simulink model "test03_mod02_firmware_removed"  (Simulink 7.3)
settings: Solver=FixedStepDiscrete  SolverMode=SingleTasking  StartTime=0.0  StopTime=inf  FixedStep=0.01  RelTol=1e-3  SampleTimeConstraint=Specified
undefined symbols (not defined in the file or in its folder): serial
libraries: simulink x6, instrumentlib x3, NAV420Lib x1
settings Model: Creator=Administrateur  LastModifiedBy=Administrateur
settings MATStruct: SampleTime=0.1  Offset=0  Priority=[10.0]

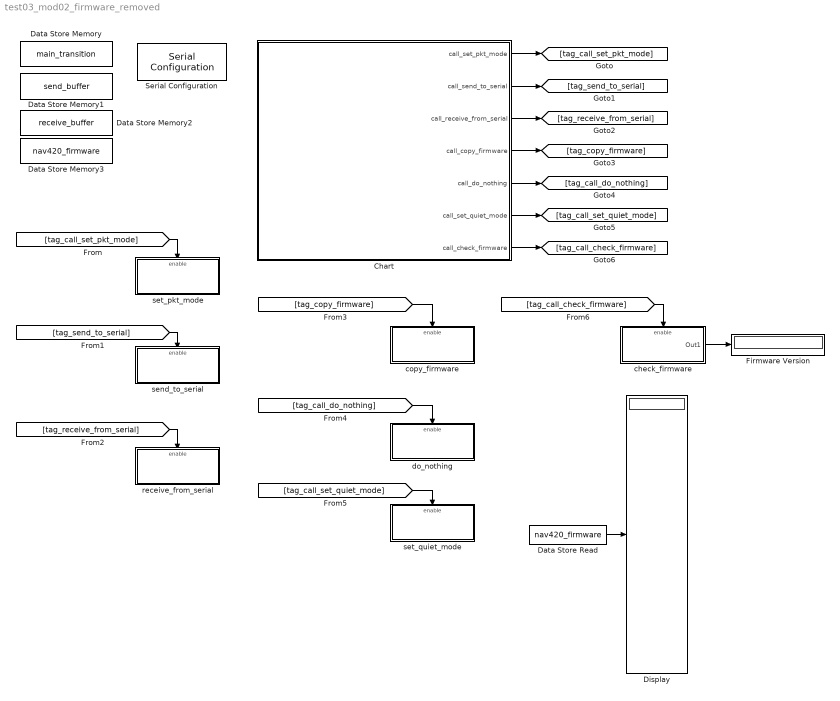
== system test03_mod02_firmware_removed ==
  Chart : Stateflow chart
  Data Store Memory : DataStoreMemory  DataStoreName=main_transition  InitialValue=0.0  DataType=double  OutDataType=fixdt(1, 16)  OutScaling=2^0  OutDataTypeStr=double
  Data Store Memory1 : DataStoreMemory  DataStoreName=send_buffer  InitialValue=[0 0 0 0 0 0 0 0 0 0 0 0 0 0 0 0 0 0 0 0 0 0 0 0 0 0 0 0 0 0 0 0 0 0 0 0 0 0 0 0]  DataType=uint8  OutDataType=fixdt(1, 16)  OutScaling=2^0  OutDataTypeStr=uint8
  Data Store Memory2 : DataStoreMemory  DataStoreName=receive_buffer  InitialValue=[0 0 0 0 0 0 0 0 0 0 0 0 0 0 0 0 0 0 0 0 0 0 0 0 0 0 0 0 0 0 0 0 0 0 0 0 0 0 0 0]  DataType=uint8  OutDataType=fixdt(1, 16)  OutScaling=2^0  OutDataTypeStr=uint8
  Data Store Memory3 : DataStoreMemory  DataStoreName=nav420_firmware  InitialValue=[0 0 0 0 0 0 0 0 0 0 0 0 0 0 0 0 0 0 0 0 0 0 0 0 0 0 0 0 0 0 0 0 0 0 0 0 0 0 0 0]  DataType=uint8  OutDataType=fixdt(1, 16)  OutScaling=2^0  OutDataTypeStr=uint8
  Data Store Read : DataStoreRead  DataStoreName=nav420_firmware  SampleTime=-1
  Display : Display
      settings: Format=hex (Stored Integer)
  Firmware Version : Display
  Serial Configuration : instrumentlib/Serial Configuration  Priority=-200000  DialogController=instrumentcreatedialog  DialogControllerArgs=DataTag0  ComPortMenu=COM4  ComPort=COM4  ObjConstructor=serial('COM4');  BaudRate=38400  DataBits=8  Parity=none  StopBits=1  FlowControl=none  Timeout=10  ByteOrder=LittleEndian
  check_firmware : Subsystem
  copy_firmware : Subsystem
  do_nothing : Subsystem
  receive_from_serial : Subsystem  TreatAsAtomicUnit=on
  send_to_serial : Subsystem  TreatAsAtomicUnit=on
  set_pkt_mode : Subsystem  TreatAsAtomicUnit=on
  set_quiet_mode : Subsystem
  wires:
  [tag_call_set_pkt_mode] -> set_pkt_mode/Enable
  [tag_send_to_serial] -> send_to_serial/Enable
  [tag_receive_from_serial] -> receive_from_serial/Enable
  [tag_copy_firmware] -> copy_firmware/Enable
  [tag_call_do_nothing] -> do_nothing/Enable
  [tag_call_set_quiet_mode] -> set_quiet_mode/Enable
  [tag_call_check_firmware] -> check_firmware/Enable
  check_firmware/1(Out1) -> Firmware Version/1
  Data Store Read/1 -> Display/1
  Chart/1(call_set_pkt_mode) -> [tag_call_set_pkt_mode]
  Chart/2(call_send_to_serial) -> [tag_send_to_serial]
  Chart/3(call_receive_from_serial) -> [tag_receive_from_serial]
  Chart/4(call_copy_firmware) -> [tag_copy_firmware]
  Chart/5(call_do_nothing) -> [tag_call_do_nothing]
  Chart/6(call_set_quiet_mode) -> [tag_call_set_quiet_mode]
  Chart/7(call_check_firmware) -> [tag_call_check_firmware]

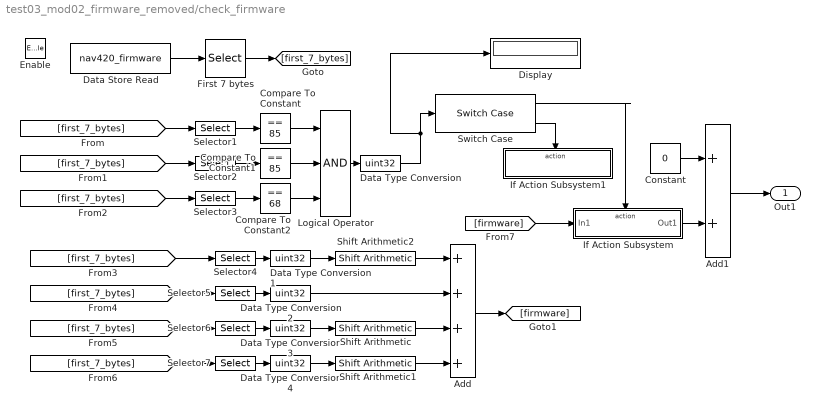
== system test03_mod02_firmware_removed/check_firmware ==
  Enable : EnablePort
  Add : Sum  Inputs=++++  AccumDataTypeStr=int32  OutDataTypeMode=int32  OutDataType=fixdt(1, 16)  OutScaling=2^-10  OutDataTypeStr=int32  InputSameDT=on
  Add1 : Sum  AccumDataTypeStr=int32  OutDataTypeMode=int32  OutDataType=fixdt(1, 16)  OutScaling=2^-10  OutDataTypeStr=int32  InputSameDT=on
  Compare To Constant : simulink/Logic and Bit Operations/Compare To Constant  SystemSampleTime=-1  relop===  const=85  LogicOutDataTypeMode=boolean  ZeroCross=off
  Compare To Constant1 : simulink/Logic and Bit Operations/Compare To Constant  SystemSampleTime=-1  relop===  const=85  LogicOutDataTypeMode=boolean  ZeroCross=off
  Compare To Constant2 : simulink/Logic and Bit Operations/Compare To Constant  SystemSampleTime=-1  relop===  const=68  LogicOutDataTypeMode=boolean  ZeroCross=off
  Constant : Constant  Value=0  OutDataTypeMode=int32  OutDataType=fixdt(1, 16)  OutScaling=2^0  OutDataTypeStr=int32  SampleTime=-1
  Data Store Read : DataStoreRead  DataStoreName=nav420_firmware  SampleTime=-1
  Data Type Conversion{,1..4} (5 alike) : DataTypeConversion  OutDataTypeMode=uint32  OutDataType=fixdt(1, 16)  OutScaling=2^0  OutDataTypeStr=uint32
  Display : Display
  First 7 bytes : Selector  InputPortWidth=40  IndexOptions=Index vector (dialog)  Indices=[1 2 3 4 5 6 7]  OutputSizes=1
  If Action Subsystem : Subsystem  TreatAsAtomicUnit=on
  If Action Subsystem1 : Subsystem  TreatAsAtomicUnit=on
  Logical Operator : Logic  Inputs=3  AllPortsSameDT=off  OutDataTypeMode=boolean  LogicDataType=fixdt(0, 8)  OutDataTypeStr=boolean
  Selector1 : Selector  InputPortWidth=7  IndexOptions=Index vector (dialog)  Indices=[1]  OutputSizes=1
  Selector2 : Selector  InputPortWidth=7  IndexOptions=Index vector (dialog)  Indices=[2]  OutputSizes=1
  Selector3 : Selector  InputPortWidth=7  IndexOptions=Index vector (dialog)  Indices=[3]  OutputSizes=1
  Selector4 : Selector  InputPortWidth=7  IndexOptions=Index vector (dialog)  Indices=[4]  OutputSizes=1
  Selector5 : Selector  InputPortWidth=7  IndexOptions=Index vector (dialog)  Indices=[5]  OutputSizes=1
  Selector6 : Selector  InputPortWidth=7  IndexOptions=Index vector (dialog)  Indices=[6]  OutputSizes=1
  Selector7 : Selector  InputPortWidth=7  IndexOptions=Index vector (dialog)  Indices=[7]  OutputSizes=1
  Shift Arithmetic : simulink/Logic and Bit Operations/Shift Arithmetic  SystemSampleTime=-1  nBitShiftRight=-24  nBinPtShiftRight=0
  Shift Arithmetic1 : simulink/Logic and Bit Operations/Shift Arithmetic  SystemSampleTime=-1  nBitShiftRight=-16  nBinPtShiftRight=0
  Shift Arithmetic2 : simulink/Logic and Bit Operations/Shift Arithmetic  SystemSampleTime=-1  nBitShiftRight=-8  nBinPtShiftRight=0
  Switch Case : SwitchCase
  Out1 : Outport  DataType=int32  OutDataType=fixdt(1, 16)  OutScaling=2^0  OutDataTypeStr=int32  InitialOutput=[0]
  wires:
  Data Store Read/1 -> First 7 bytes/1
  First 7 bytes/1 -> [first_7_bytes]
  [first_7_bytes] -> Selector1/1
  Selector1/1 -> Compare To Constant/1
  [first_7_bytes] -> Selector2/1
  Selector2/1 -> Compare To Constant1/1
  [first_7_bytes] -> Selector3/1
  Selector3/1 -> Compare To Constant2/1
  Compare To Constant2/1 -> Logical Operator/3
  Compare To Constant1/1 -> Logical Operator/2
  Compare To Constant/1 -> Logical Operator/1
  Logical Operator/1 -> Data Type Conversion/1
  Data Type Conversion/1 -> Switch Case/1, Display/1
  Switch Case/1 -> If Action Subsystem/Action
  [first_7_bytes] -> Selector4/1
  [first_7_bytes] -> Selector5/1
  [first_7_bytes] -> Selector6/1
  [first_7_bytes] -> Selector7/1
  Data Type Conversion2/1 -> Add/2
  Shift Arithmetic2/1 -> Add/1
  Shift Arithmetic/1 -> Add/3
  Shift Arithmetic1/1 -> Add/4
  Data Type Conversion4/1 -> Shift Arithmetic1/1
  Data Type Conversion3/1 -> Shift Arithmetic/1
  Data Type Conversion1/1 -> Shift Arithmetic2/1
  Selector4/1 -> Data Type Conversion1/1
  Selector5/1 -> Data Type Conversion2/1
  Selector6/1 -> Data Type Conversion3/1
  Selector7/1 -> Data Type Conversion4/1
  Add/1 -> [firmware]
  [firmware] -> If Action Subsystem/1(In1)
  If Action Subsystem/1(Out1) -> Add1/2
  Constant/1 -> Add1/1
  Add1/1 -> Out1/1
  Switch Case/2 -> If Action Subsystem1/Action

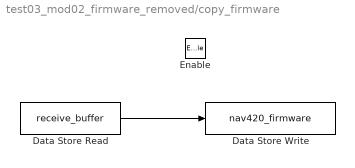
== system test03_mod02_firmware_removed/copy_firmware ==
  Enable : EnablePort
  Data Store Read : DataStoreRead  DataStoreName=receive_buffer  SampleTime=-1
  Data Store Write : DataStoreWrite  DataStoreName=nav420_firmware  SampleTime=-1
  wires:
  Data Store Read/1 -> Data Store Write/1

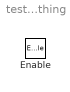
== system test03_mod02_firmware_removed/do_nothing ==
  Enable : EnablePort

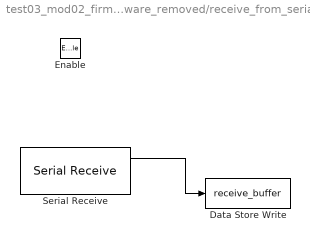
== system test03_mod02_firmware_removed/receive_from_serial ==
  Enable : EnablePort
  Data Store Write : DataStoreWrite  DataStoreName=receive_buffer  SampleTime=-1
  Serial Receive : instrumentlib/Serial Receive  DialogController=instrumentcreatedialog  DialogControllerArgs=DataTag1  ComPortMenu=COM4  ComPort=COM4  ObjConstructor=serial('COM4');  Terminator=<none>  DataSize="[40   1]"  DataType=uint8  EnableBlockingMode=off  ActionDataUnavailable=Output last received value  CustomValue=0  SampleTime=-1
  wires:
  Serial Receive/1 -> Data Store Write/1

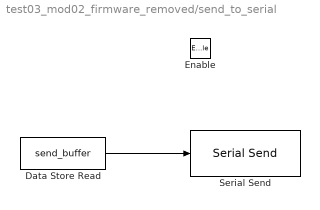
== system test03_mod02_firmware_removed/send_to_serial ==
  Enable : EnablePort
  Data Store Read : DataStoreRead  DataStoreName=send_buffer  SampleTime=-1
  Serial Send : instrumentlib/Serial Send  DialogController=instrumentcreatedialog  DialogControllerArgs=DataTag2  ComPortMenu=COM4  ComPort=COM4  ObjConstructor=serial('COM4');  Terminator=<none>  EnableBlockingMode=off
  wires:
  Data Store Read/1 -> Serial Send/1

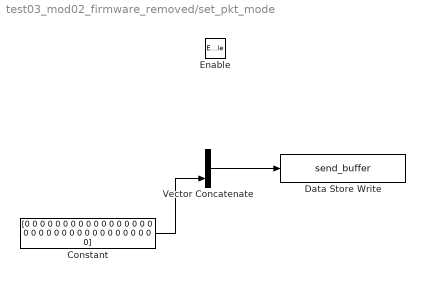
== system test03_mod02_firmware_removed/set_pkt_mode ==
  Enable : EnablePort
  Constant : Constant  Value=[0 0 0 0 0 0 0 0 0 0 0 0 0 0 0 0 0 0 0 0 0 0 0 0 0 0 0 0 0 0 0 0 0 0 0]  OutDataTypeMode=uint8  OutDataType=fixdt(1, 16)  OutScaling=2^0  OutDataTypeStr=uint8  SampleTime=-1
  Data Store Write : DataStoreWrite  DataStoreName=send_buffer  SampleTime=-1
  Vector Concatenate : Concatenate  Mode=Vector
  wires:
  ? -> Vector Concatenate/1
  Constant/1 -> Vector Concatenate/2
  Vector Concatenate/1 -> Data Store Write/1

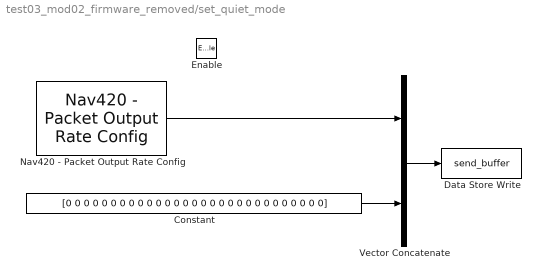
== system test03_mod02_firmware_removed/set_quiet_mode ==
  Enable : EnablePort
  Constant : Constant  Value=[0 0 0 0 0 0 0 0 0 0 0 0 0 0 0 0 0 0 0 0 0 0 0 0 0 0 0 0 0]  OutDataTypeMode=uint8  OutDataType=fixdt(1, 16)  OutScaling=2^0  OutDataTypeStr=uint8  SampleTime=-1
  Data Store Write : DataStoreWrite  DataStoreName=send_buffer  SampleTime=-1
  Nav420 - Packet Output Rate Config : NAV420Lib/Nav420 - Packet Output Rate Config  SystemSampleTime=-1  shouldSave=on  output_rate=0
  Vector Concatenate : Concatenate  Mode=Vector
  wires:
  Constant/1 -> Vector Concatenate/2
  Nav420 - Packet Output Rate Config/1 -> Vector Concatenate/1
  Vector Concatenate/1 -> Data Store Write/1

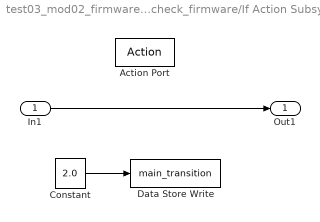
== system test03_mod02_firmware_removed/check_firmware/If Action Subsystem ==
  In1 : Inport  DataType=int32  OutDataType=fixdt(1, 16)  OutScaling=2^0  OutDataTypeStr=int32
  Action Port : ActionPort  ActionType=case
  Constant : Constant  Value=2.0  OutDataTypeMode=double  OutDataType=fixdt(1, 16)  OutScaling=2^0  OutDataTypeStr=double  SampleTime=-1
  Data Store Write : DataStoreWrite  DataStoreName=main_transition  SampleTime=-1
  Out1 : Outport  OutDataType=fixdt(1, 16)  OutScaling=2^0  OutputWhenDisabled=reset  InitialOutput=[0]
  wires:
  In1/1 -> Out1/1
  Constant/1 -> Data Store Write/1

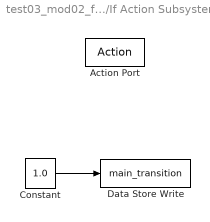
== system test03_mod02_firmware_removed/check_firmware/If Action Subsystem1 ==
  Action Port : ActionPort  ActionType=default
  Constant : Constant  Value=1.0  OutDataTypeMode=double  OutDataType=fixdt(1, 16)  OutScaling=2^0  OutDataTypeStr=double  SampleTime=-1
  Data Store Write : DataStoreWrite  DataStoreName=main_transition  SampleTime=-1
  wires:
  Constant/1 -> Data Store Write/1

== stateflow chart Chart ==
  state Request_Serial
    call_set_pkt_mode=1;
    call_send_to_serial=1;
    call_receive_from_serial=1;
    call_copy_firmware=1;
    call_check_firmware=1;
  state Be_Idle
    call_do_nothing=1;
  state Set_Quiet_Mode
    main_transition=1.0;
    call_set_quiet_mode=1;
    call_send_to_serial=1;
  Request_Serial -> Be_Idle [order 1] : [main_transition==2.0]
  Set_Quiet_Mode -> Request_Serial : [main_transition==1.0]
  (default) -> Set_Quiet_Mode
  Request_Serial -> Set_Quiet_Mode [order 2] : [main_transition==1.0]
  data: main_transition data_store_memory double; call_set_pkt_mode output double; call_send_to_serial output double; call_receive_from_serial output double; call_copy_firmware output double; call_do_nothing output double; call_set_quiet_mode output double; call_check_firmware output double
